simulink model "Get_RE_RhythmCalc_Sig2Mbed_plotdTdAV2"  (R2013a)
settings: Solver=FixedStepDiscrete  StartTime=0.0  StopTime=60  RelTol=1e-3
undefined symbols (not defined in the file): ts
libraries: arduino_io_lib x12, simulink x4
settings Model: Creator=cell  LastModifiedBy=cell
settings OptimizationCC: OptimizeModelRefInitCode=on  LifeSpan=1
settings DebuggingCC: InheritedTsInSrcMsg=none  StrictBusMsg=Warning
settings HardwareCC: ProdBitPerInt=16  ProdBitPerPointer=8  ProdIntDivRoundTo=Zero  ProdEndianess=LittleEndian  ProdWordSize=8  ProdHWDeviceType=Atmel->AVR
settings RTWCC: SystemTargetFile=realtime.tlc  GenerateMakefile=off  TemplateMakefile=realtime.tmf  Description=Run on Target Hardware  RTWVerbose=off  ProcessScript=realtime_make_rtw_hook
settings CodeAppCC: IgnoreCustomStorageClasses=off
settings STFCustomTargetCC: TargetLibSuffix=.a  GenerateSampleERTMain=on  CombineOutputUpdateFcns=on  ERTCustomFileBanners=on  SupportContinuousTime=off  SupportNonInlinedSFcns=off  MATLABClassNameForMDSCustomization=Simulink.SoftwareTarget.ERTCustomization  SystemTargetFile=realtime.tlc
settings ERTTargetCC: ParMdlRefBuildCompliant=off  CompOptLevelCompliant=off  ConcurrentExecutionCompliant=off  ERTFirstTimeCompliant=off  ModelStepFunctionPrototypeControlCompliant=off  CPPClassGenCompliant=off  ERTCustomFileTemplate=realtime_file_process.tlc

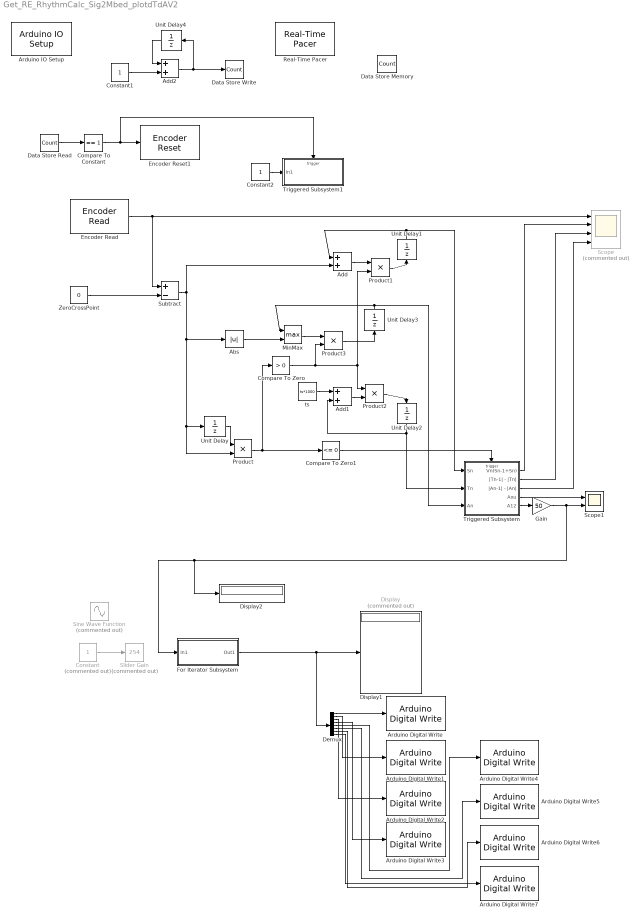
== system Get_RE_RhythmCalc_Sig2Mbed_plotdTdAV2 ==
  Abs : Abs
  Add : Sum
  Add1 : Sum
  Add2 : Sum
  Arduino Digital Write : arduino_io_lib/Arduino Digital Write  arduinoVar=Existing workspace arduino variable #1  arduinoPin=6  T=ts
  Arduino Digital Write1 : arduino_io_lib/Arduino Digital Write  arduinoVar=Existing workspace arduino variable #1  arduinoPin=7  T=ts
  Arduino Digital Write2 : arduino_io_lib/Arduino Digital Write  arduinoVar=Existing workspace arduino variable #1  arduinoPin=8  T=ts
  Arduino Digital Write3 : arduino_io_lib/Arduino Digital Write  arduinoVar=Existing workspace arduino variable #1  arduinoPin=9  T=ts
  Arduino Digital Write4 : arduino_io_lib/Arduino Digital Write  arduinoVar=Existing workspace arduino variable #1  arduinoPin=10  T=ts
  Arduino Digital Write5 : arduino_io_lib/Arduino Digital Write  arduinoVar=Existing workspace arduino variable #1  arduinoPin=11  T=ts
  Arduino Digital Write6 : arduino_io_lib/Arduino Digital Write  arduinoVar=Existing workspace arduino variable #1  arduinoPin=12  T=ts
  Arduino Digital Write7 : arduino_io_lib/Arduino Digital Write  arduinoVar=Existing workspace arduino variable #1  arduinoPin=13  T=ts
  Arduino IO Setup : arduino_io_lib/Arduino IO Setup  Priority=3  arduinoVar=Existing workspace arduino variable #1  workspaceVarName=a  comPort=DEMO
  Compare To Constant : simulink/Logic and Bit Operations/Compare To Constant  relop===  const=1  OutDataTypeStr=boolean
  Compare To Zero : simulink/Logic and Bit Operations/Compare To Zero  relop=>  OutDataTypeStr=boolean
  Compare To Zero1 : simulink/Logic and Bit Operations/Compare To Zero  relop=<=  OutDataTypeStr=boolean
  Constant : Constant  Commented=on
  Constant1 : Constant
  Constant2 : Constant
  Data Store Memory : DataStoreMemory  DataStoreName=Count  ReadBeforeWriteMsg=warning  WriteAfterWriteMsg=warning  WriteAfterReadMsg=warning
  Data Store Read : DataStoreRead  DataStoreName=Count
  Data Store Write : DataStoreWrite  DataStoreName=Count
  Demux : Demux  Outputs=8
  Display : Display  Commented=on
  Display1 : Display
  Display2 : Display
  Encoder Read : arduino_io_lib/Encoder Read  arduinoVar=Existing workspace arduino variable #1  encNum=1  pinA=2  pinB=3  DbDl=0  T=ts
  Encoder Reset1 : arduino_io_lib/Encoder Reset  arduinoVar=Existing workspace arduino variable #1  encNum=1  T=ts
  For Iterator Subsystem : Subsystem  TreatAsAtomicUnit=on  mask{bits=8}
      mask prompts: bits "ビット数"
      mask Display: disp('Integer To Bit\nConvertor')
  Gain : Gain  Gain=50
  MinMax : MinMax  Function=max  Inputs=2  OutDataTypeStr=double
      settings: LockScale=on
  Product{,1..3} (4 alike) : Product
  Real-Time Pacer : arduino_io_lib/Real-Time Pacer  simTimePerRealTime=1
  Scope : Scope  Commented=on  NumInputPorts=4
      settings: TimeRange=10  YMin=-50~-250~0~0  YMax=225~2500~4000~140
  Scope1 : Scope  NumInputPorts=2
      settings: YMin=-25~0  YMax=2.5~70
  Sine Wave Function : Sin  Commented=on  SineType=Sample based  Amplitude=100  Bias=100  Samples=80  SampleTime=ts
  Slider Gain : simulink/Math Operations/Slider Gain  Commented=on  low=0  gain=254  high=254
  Subtract : Sum  Inputs=+-
  Triggered Subsystem : Subsystem  TreatAsAtomicUnit=on
  Triggered Subsystem1 : Subsystem  TreatAsAtomicUnit=on
  Unit Delay{,1..4} (5 alike) : UnitDelay  SampleTime=-1
  ZeroCrossPoint : Constant  Value=0
  ts : Constant  Value=ts*1000
  wires:
  Encoder Read/1 -> Subtract/1, Scope/1
  For Iterator Subsystem/1(Out1) -> Display1/1, Demux/1
  Demux/1 -> Arduino Digital Write/1
  Demux/2 -> Arduino Digital Write1/1
  Demux/3 -> Arduino Digital Write2/1
  Demux/4 -> Arduino Digital Write3/1
  Demux/5 -> Arduino Digital Write4/1
  Demux/6 -> Arduino Digital Write5/1
  Demux/7 -> Arduino Digital Write6/1
  Demux/8 -> Arduino Digital Write7/1
  Unit Delay/1 -> Product/1
  ZeroCrossPoint/1 -> Subtract/2
  Compare To Zero1/1 -> Triggered Subsystem/Trigger
  Product/1 -> Compare To Zero1/1, Compare To Zero/1
  Subtract/1 -> Product/2, Unit Delay/1, Abs/1, Add/2
  Product1/1 -> Unit Delay1/1
  Constant/1 -> Slider Gain/1
  Compare To Zero/1 -> Product3/2, Product1/2, Product2/1
  Unit Delay2/1 -> Add1/2, Triggered Subsystem/2(Tn)
  Add1/1 -> Product2/2
  Product2/1 -> Unit Delay2/1
  ts/1 -> Add1/1
  Unit Delay1/1 -> Triggered Subsystem/1(Sn), Add/1
  Add/1 -> Product1/1
  Abs/1 -> MinMax/2
  Triggered Subsystem/3(|An-1| - |An|) -> Scope/4
  MinMax/1 -> Product3/1
  Product3/1 -> Unit Delay3/1
  Constant1/1 -> Add2/2
  Add2/1 -> Data Store Write/1, Unit Delay4/1
  Triggered Subsystem/1(Vn(Sn-1+Sn)) -> Scope/2
  Triggered Subsystem/2(|Tn-1| - |Tn|) -> Scope/3
  Unit Delay3/1 -> MinMax/1, Triggered Subsystem/3(An)
  Unit Delay4/1 -> Add2/1
  Data Store Read/1 -> Compare To Constant/1
  Compare To Constant/1 -> Triggered Subsystem1/Trigger, Encoder Reset1/1
  Triggered Subsystem/4(Axu) -> Scope1/1
  Constant2/1 -> Triggered Subsystem1/1(In1)
  Triggered Subsystem/5(A12) -> Gain/1
  Gain/1 -> Display2/1, For Iterator Subsystem/1(In1), Scope1/2

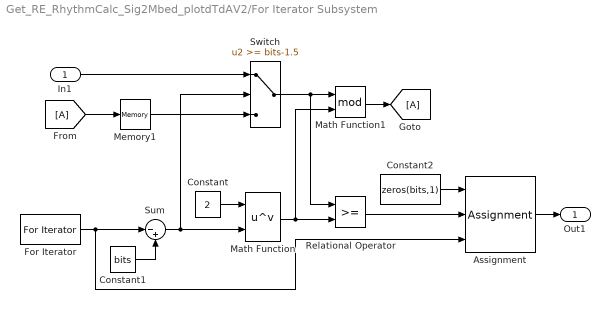
== system Get_RE_RhythmCalc_Sig2Mbed_plotdTdAV2/For Iterator Subsystem ==
  In1 : Inport
  Assignment : Assignment  IndexOptions=Index vector (port)  Indices=1  OutputSizes=[1 1]
  Constant : Constant  Value=2
  Constant1 : Constant  Value=bits
  Constant2 : Constant  Value=zeros(bits,1)  VectorParams1D=off
  For Iterator : ForIterator  IterationLimit=bits
  Math Function : Math  Operator=pow  SaturateOnIntegerOverflow=on
  Math Function1 : Math  Operator=mod  SaturateOnIntegerOverflow=on
  Memory1 : Memory  InheritSampleTime=on
  Relational Operator : RelationalOperator  OutDataTypeStr=float('double')
  Sum : Sum  Inputs=|-+
  Switch : Switch  Threshold=bits-1.5
  Out1 : Outport
  wires:
  For Iterator/1 -> Sum/1, Assignment/3
  Constant/1 -> Math Function/1
  Sum/1 -> Math Function/2, Switch/2
  Constant1/1 -> Sum/2
  Math Function/1 -> Math Function1/2, Relational Operator/2
  Switch/1 -> Math Function1/1, Relational Operator/1
  In1/1 -> Switch/1
  Memory1/1 -> Switch/3
  Assignment/1 -> Out1/1
  Constant2/1 -> Assignment/1
  Relational Operator/1 -> Assignment/2
  [A] -> Memory1/1
  Math Function1/1 -> [A]

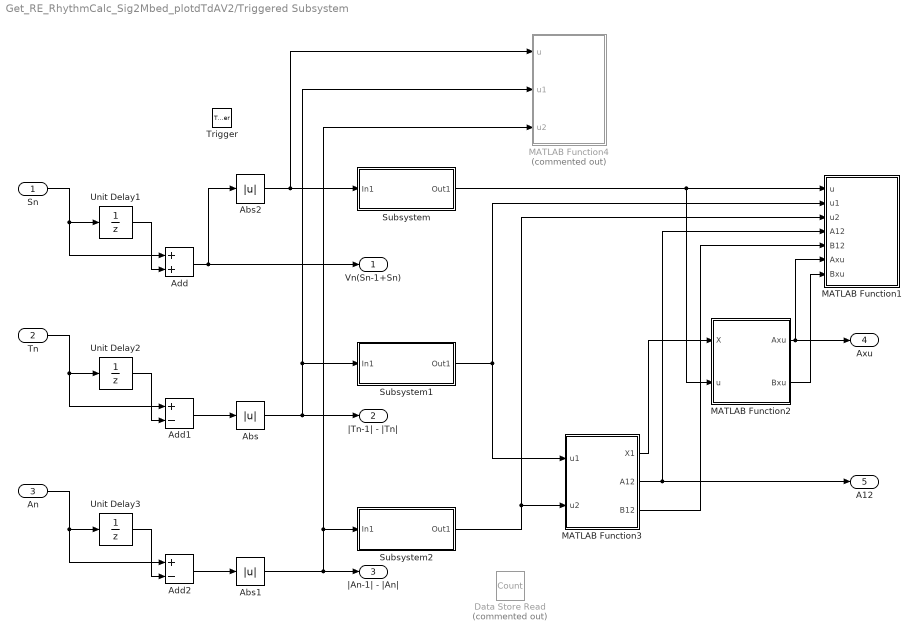
== system Get_RE_RhythmCalc_Sig2Mbed_plotdTdAV2/Triggered Subsystem ==
  Sn : Inport
  Tn : Inport  Port=2
  An : Inport  Port=3
  Trigger : TriggerPort
  Abs : Abs
  Abs1 : Abs
  Abs2 : Abs
  Add : Sum
  Add1 : Sum  Inputs=+-
  Add2 : Sum  Inputs=+-
  Data Store Read : DataStoreRead  Commented=on  DataStoreName=Count
  MATLAB Function1 : MATLAB Function  TreatAsAtomicUnit=on
  MATLAB Function2 : MATLAB Function  TreatAsAtomicUnit=on
  MATLAB Function3 : MATLAB Function  TreatAsAtomicUnit=on
  MATLAB Function4 : MATLAB Function  Commented=on  TreatAsAtomicUnit=on
  Subsystem : Subsystem
  Subsystem1 : Subsystem
  Subsystem2 : Subsystem
  Unit Delay1 : UnitDelay  SampleTime=-1
  Unit Delay2 : UnitDelay  SampleTime=-1
  Unit Delay3 : UnitDelay  SampleTime=-1
  Vn(Sn-1+Sn) : Outport
  |Tn-1| - |Tn| : Outport  Port=2
  |An-1| - |An| : Outport  Port=3
  Axu : Outport  Port=4
  A12 : Outport  Port=5
  wires:
  Unit Delay1/1 -> Add/2
  Sn/1 -> Add/1, Unit Delay1/1
  Unit Delay2/1 -> Add1/2
  Tn/1 -> Add1/1, Unit Delay2/1
  Add1/1 -> Abs/1
  Unit Delay3/1 -> Add2/2
  An/1 -> Unit Delay3/1, Add2/1
  Add2/1 -> Abs1/1
  Abs1/1 -> MATLAB Function4/3(u2), Subsystem2/1(In1), |An-1| - |An|/1
  Add/1 -> Abs2/1, Vn(Sn-1+Sn)/1
  Abs/1 -> Subsystem1/1(In1), MATLAB Function4/2(u1), |Tn-1| - |Tn|/1
  Abs2/1 -> MATLAB Function4/1(u), Subsystem/1(In1)
  Subsystem1/1(Out1) -> MATLAB Function1/2(u1), MATLAB Function3/1(u1)
  Subsystem2/1(Out1) -> MATLAB Function1/3(u2), MATLAB Function3/2(u2)
  MATLAB Function3/1(X1) -> MATLAB Function2/1(X)
  Subsystem/1(Out1) -> MATLAB Function1/1(u), MATLAB Function2/2(u)
  MATLAB Function2/1(Axu) -> MATLAB Function1/6(Axu), Axu/1
  MATLAB Function2/2(Bxu) -> MATLAB Function1/7(Bxu)
  MATLAB Function3/3(B12) -> MATLAB Function1/5(B12)
  MATLAB Function3/2(A12) -> MATLAB Function1/4(A12), A12/1

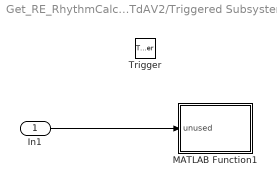
== system Get_RE_RhythmCalc_Sig2Mbed_plotdTdAV2/Triggered Subsystem1 ==
  In1 : Inport
  Trigger : TriggerPort
  MATLAB Function1 : MATLAB Function  TreatAsAtomicUnit=on
  wires:
  In1/1 -> MATLAB Function1/1(unused)

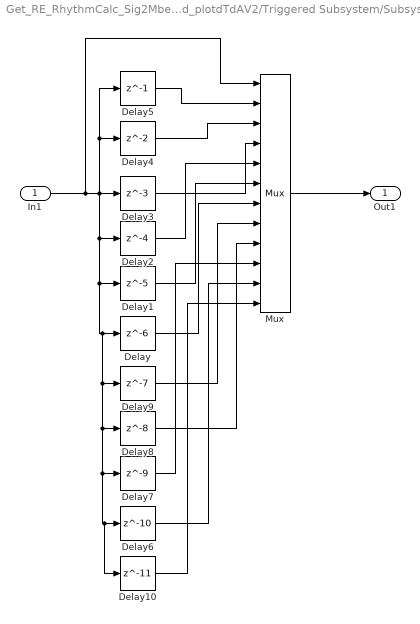
== system Get_RE_RhythmCalc_Sig2Mbed_plotdTdAV2/Triggered Subsystem/Subsystem ==
  In1 : Inport
  Delay : Delay  DelayLength=6
  Delay1 : Delay  DelayLength=5
  Delay10 : Delay  DelayLength=11
  Delay2 : Delay  DelayLength=4
  Delay3 : Delay  DelayLength=3
  Delay4 : Delay
  Delay5 : Delay  DelayLength=1
  Delay6 : Delay  DelayLength=10
  Delay7 : Delay  DelayLength=9
  Delay8 : Delay  DelayLength=8
  Delay9 : Delay  DelayLength=7
  Mux : Mux  Inputs=12
  Out1 : Outport
  wires:
  In1/1 -> Delay5/1, Delay4/1, Delay10/1, Delay6/1, Delay7/1, Delay8/1, Delay9/1, Delay/1, Delay1/1, Delay2/1, Delay3/1, Mux/1
  Delay5/1 -> Mux/2
  Delay4/1 -> Mux/3
  Delay3/1 -> Mux/4
  Delay2/1 -> Mux/5
  Delay1/1 -> Mux/6
  Delay/1 -> Mux/7
  Mux/1 -> Out1/1
  Delay9/1 -> Mux/8
  Delay8/1 -> Mux/9
  Delay7/1 -> Mux/10
  Delay6/1 -> Mux/11
  Delay10/1 -> Mux/12

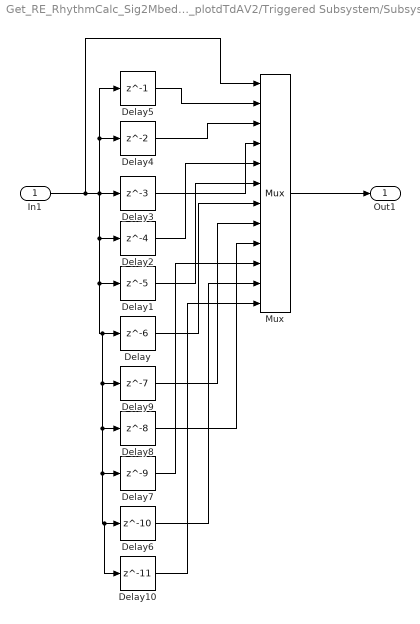
== system Get_RE_RhythmCalc_Sig2Mbed_plotdTdAV2/Triggered Subsystem/Subsystem1 ==
  In1 : Inport
  Delay : Delay  DelayLength=6
  Delay1 : Delay  DelayLength=5
  Delay10 : Delay  DelayLength=11
  Delay2 : Delay  DelayLength=4
  Delay3 : Delay  DelayLength=3
  Delay4 : Delay
  Delay5 : Delay  DelayLength=1
  Delay6 : Delay  DelayLength=10
  Delay7 : Delay  DelayLength=9
  Delay8 : Delay  DelayLength=8
  Delay9 : Delay  DelayLength=7
  Mux : Mux  Inputs=12
  Out1 : Outport
  wires:
  Delay10/1 -> Mux/12
  Delay6/1 -> Mux/11
  Delay7/1 -> Mux/10
  Delay8/1 -> Mux/9
  Delay9/1 -> Mux/8
  Mux/1 -> Out1/1
  Delay/1 -> Mux/7
  Delay1/1 -> Mux/6
  Delay2/1 -> Mux/5
  Delay3/1 -> Mux/4
  Delay4/1 -> Mux/3
  Delay5/1 -> Mux/2
  In1/1 -> Mux/1, Delay3/1, Delay2/1, Delay1/1, Delay/1, Delay9/1, Delay8/1, Delay7/1, Delay6/1, Delay10/1, Delay4/1, Delay5/1

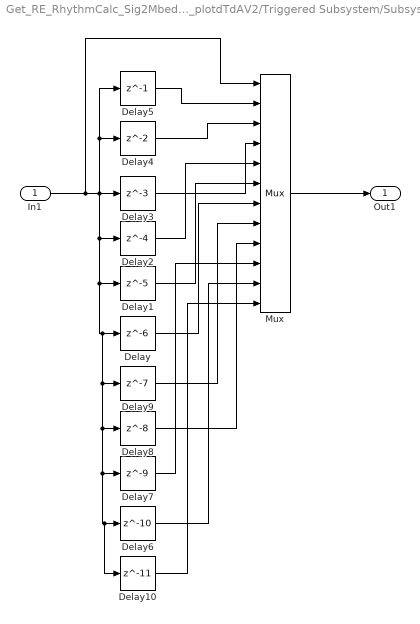
== system Get_RE_RhythmCalc_Sig2Mbed_plotdTdAV2/Triggered Subsystem/Subsystem2 ==
  In1 : Inport
  Delay : Delay  DelayLength=6
  Delay1 : Delay  DelayLength=5
  Delay10 : Delay  DelayLength=11
  Delay2 : Delay  DelayLength=4
  Delay3 : Delay  DelayLength=3
  Delay4 : Delay
  Delay5 : Delay  DelayLength=1
  Delay6 : Delay  DelayLength=10
  Delay7 : Delay  DelayLength=9
  Delay8 : Delay  DelayLength=8
  Delay9 : Delay  DelayLength=7
  Mux : Mux  Inputs=12
  Out1 : Outport
  wires:
  In1/1 -> Delay5/1, Delay4/1, Delay10/1, Delay6/1, Delay7/1, Delay8/1, Delay9/1, Delay/1, Delay1/1, Delay2/1, Delay3/1, Mux/1
  Delay5/1 -> Mux/2
  Delay4/1 -> Mux/3
  Delay3/1 -> Mux/4
  Delay2/1 -> Mux/5
  Delay1/1 -> Mux/6
  Delay/1 -> Mux/7
  Mux/1 -> Out1/1
  Delay9/1 -> Mux/8
  Delay8/1 -> Mux/9
  Delay7/1 -> Mux/10
  Delay6/1 -> Mux/11
  Delay10/1 -> Mux/12

== matlab function Get_RE_RhythmCalc_Sig2Mbed_plotdTdAV2/Triggered Subsystem1/MATLAB Function1 ==
  data: unused input
function initPlot(~)
%#codegen

figure(1)
clf
MonitorSize = [ 0, 0, 500, 500];
set(gcf, 'Position', MonitorSize);

plot3( 0, 0 , 0 , '.','MarkerSize',1);
grid on
axis square
view(-30,25);
xlim([0 600]);            ylim([0 600]);          zlim([0 5000]);
xlabel('dT');    ylabel('dA’');

== matlab function Get_RE_RhythmCalc_Sig2Mbed_plotdTdAV2/Triggered Subsystem/MATLAB Function2 ==
  data: X input; u input; Axu output; Bxu output
function [ Axu , Bxu]  = ols_method2( X, u )
%#codegen

% coder.extrinsic('polyfit')
    
% if length(u1) == 7
%     [au12 , bu12]= polyfit(u1 , u2 , 1);
% end

% if Count ==1
%     Sx = sum(u1(1:end-1));
%     Sy = sum(u2(1:end-1));
%     Sxx = sum(u1(1:end-1) .* u1(1:end-1));
%     Sxy = sum( u1(1:end-1) .* u2(1:end-1));
% end

n = length(u);

Sx = sum(X);
Su = sum(u);
Sxx = sum(X .* X);
Sxu = sum(u .* X);

Axu = ( n*Sxu - Sx*Su ) / ( n*Sxx- Sx^2 );

% k1 =  1 / sqrt(1+Axu^2);    k2 = Axu / sqrt(1+Axu^2);
Bxu = ( Sxx * Su - Sxu * Sx ) / ( n*Sxx- Sx^2 );

%     pxv =  polyfit(X1, u);
 
%     Vmin =  polyval( pxv, min(X1) ) ;
%     Vmax =  polyva( pxv, max(X1) ) ;
% 
%     Rotate_inv = [ cos(-theta) sin(-theta); -sin(-theta) cos(-theta)];      % 逆回転行列
%     m1 =Rotate_inv(1,1);    m2 = Rotate_inv(1,2);
%     u1min = m1 * X1min ; %dT
%     u1max = m1 * X1min ; %dT
%     u2min = n1 * X1min ; %dA
%     u2max = n1 * X1min ; %dA
    
%     plot3( u ,u1,u2-buv, 'o','MarkerSize',2);
%     hold on
%         plot3( [0,600*k1]  , [0,600*k2] , [0,0] ,'r' );
%         plot3( [u1min u1max]  , [u2min u2max] , [Vmin Vmax] ,'r' ,'LineWidth',3 );
%         plot3( [u1max u1max] , [u2max u2max] , [0 Vmax] ,'--r' );
%     hold off

% end

== matlab function Get_RE_RhythmCalc_Sig2Mbed_plotdTdAV2/Triggered Subsystem/MATLAB Function4 ==
  data: u input; u1 input; u2 input
function  rhythmPlot( u, u1, u2  )
%#codegen

hold on
plot3( u1,u2, u,  'o','MarkerSize',2);
grid on
axis square
view(-30,25);
xlim([0 600]);            ylim([0 600]);          zlim([0 5000]);
xlabel('dT');    ylabel('dA’');

== matlab function Get_RE_RhythmCalc_Sig2Mbed_plotdTdAV2/Triggered Subsystem/MATLAB Function1 ==
  data: u input; u1 input; u2 input; A12 input; B12 input; Axu input; Bxu input
function  rhythmPlot_regress( u, u1, u2 , A12, B12 , Axu , Bxu )
%#codegen

plot3( u1,u2, u,  'o','MarkerSize',2);
k1 =  1 / sqrt(1+A12^2);    k2 = A12 / sqrt(1+A12^2);
X1max= max( k1*u1 + k2*(u2-B12) );
hold on
plot3( 500*[0 k1] , 500*[0 k2] + B12, [0 0], 'r');
plot3( [0 X1max*k1] ,[0 X1max*k2]+B12 ,[0 Axu*X1max]+Bxu  ,'r' ,'LineWidth',3 );
hold off
grid on
axis square
view(-30,25);
xlim([0 600]);            ylim([0 600]);          zlim([0 5000]);
xlabel('dT');    ylabel('dA’');

== matlab function Get_RE_RhythmCalc_Sig2Mbed_plotdTdAV2/Triggered Subsystem/MATLAB Function3 ==
  data: u1 input; u2 input; X1 output; A12 output; B12 output
% function X1   = ols_method1( Sx, Sy, Sxx, Sxy, u1, u2 , Count)
function [ X1 , A12 , B12 ]  = ols_method1( u1, u2 )
%#codegen

% coder.extrinsic('polyfit')
    
% if length(u1) == 7
%     [au12 , bu12]= polyfit(u1 , u2 , 1);
% end

% if Count ==1
%     Sx = sum(u1(1:end-1));
%     Sy = sum(u2(1:end-1));
%     Sxx = sum(u1(1:end-1) .* u1(1:end-1));
%     Sxy = sum( u1(1:end-1) .* u2(1:end-1));
% end

n = length(u1);

S1 = sum(u1);
S2 = sum(u2);
S11 = sum(u1 .* u1);
S12 = sum(u1 .* u2);

A12 = ( n*S12 - S1*S2 ) / ( n*S11- S1^2 );

k1 =  1 / sqrt(1+A12^2);    k2 = A12 / sqrt(1+A12^2);
B12 = ( S11 * S2 - S12 * S1 ) / ( n*S11- S1^2 );
X1 = k1 * u1 + k2 * (u2 - B12);

%     pxv =  polyfit(X1, u);
 
%     Vmin =  polyval( pxv, min(X1) ) ;
%     Vmax =  polyva( pxv, max(X1) ) ;
% 
%     Rotate_inv = [ cos(-theta) sin(-theta); -sin(-theta) cos(-theta)];      % 逆回転行列
%     m1 =Rotate_inv(1,1);    m2 = Rotate_inv(1,2);
%     u1min = m1 * X1min ; %dT
%     u1max = m1 * X1min ; %dT
%     u2min = n1 * X1min ; %dA
%     u2max = n1 * X1min ; %dA
    
%     plot3( u ,u1,u2-buv, 'o','MarkerSize',2);
%     hold on
%         plot3( [0,600*k1]  , [0,600*k2] , [0,0] ,'r' );
%         plot3( [u1min u1max]  , [u2min u2max] , [Vmin Vmax] ,'r' ,'LineWidth',3 );
%         plot3( [u1max u1max] , [u2max u2max] , [0 Vmax] ,'--r' );
%     hold off

% end
